simulink model "gps"  (R2015a)
settings: Solver=ode45  StartTime=0.0  StopTime=100  RelTol=1e-3
undefined symbols (not defined in the file): gpsNoise
libraries: simulink x1, dsparch4 x1
settings Model: Creator=johnz  LastModifiedBy=johnz

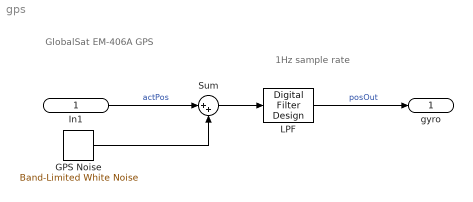
== system gps ==
  note: GlobalSat EM-406A GPS
  note: 1Hz sample rate
  In1 : Inport
  GPS Noise : simulink/Sources/Band-Limited White Noise  Cov=[gpsNoise]  Ts=1  seed=1001
  "LPF " : dsparch4/Digital Filter Design  mwdsp_browser_bugfix_var=off
  Sum : Sum  Inputs=|++
  gyro : Outport  OutDataTypeStr=double  PortDimensions=1
  wires:
  In1/1 -> Sum/1  "actPos"
  Sum/1 -> "LPF "/1
  "LPF "/1 -> gyro/1  "posOut"
  GPS Noise/1 -> Sum/2
